simulink model "model"  (R2020b)
settings: Solver=VariableStepAuto  StartTime=0.0  StopTime=100.0  RelTol=1e-3
values from neighbouring files (symbols this model uses):
  k = 100    [runme.m]
  state0 = [1;0;0]    [runme.m]
settings Model: Creator=fulvioforni  LastModifiedBy=fulvioforni

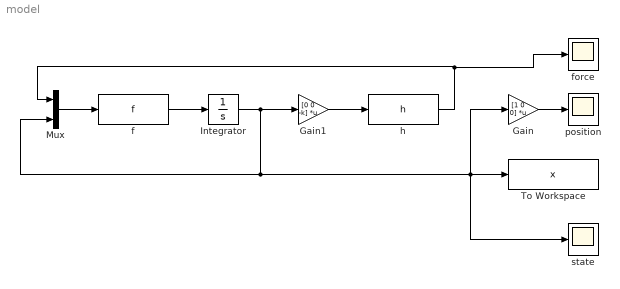
== system model ==
  Gain : Gain  Gain=[1 0 0]  Multiplication=Matrix(K*u)
  Gain1 : Gain  Gain=[0 0 -k]  Multiplication=Matrix(K*u)
  Integrator : Integrator  InitialCondition=state0
  Mux : Mux  Inputs=2
  To Workspace : ToWorkspace  VariableName=x  SaveFormat=Timeseries  SampleTime=-1
  f : MATLABFcn  MATLABFcn=f
  force : Scope
  h : MATLABFcn  MATLABFcn=h
  position : Scope
  state : Scope
  wires:
  f/1 -> Integrator/1
  Integrator/1 -> Gain1/1, state/1, Gain/1, To Workspace/1, Mux/2
  Mux/1 -> f/1
  Gain/1 -> position/1
  h/1 -> force/1, Mux/1
  Gain1/1 -> h/1
